simulink model "SM_smallScalePS"  (R2019a)
settings: Solver=ode23  StartTime=0.0  StopTime=5  RelTol=1e-3
undefined symbols (not defined in the file): D1, Delta
libraries: powerlib x9, sps_avr x1, spsHTGModel x1
settings Model: Creator=User  LastModifiedBy=User

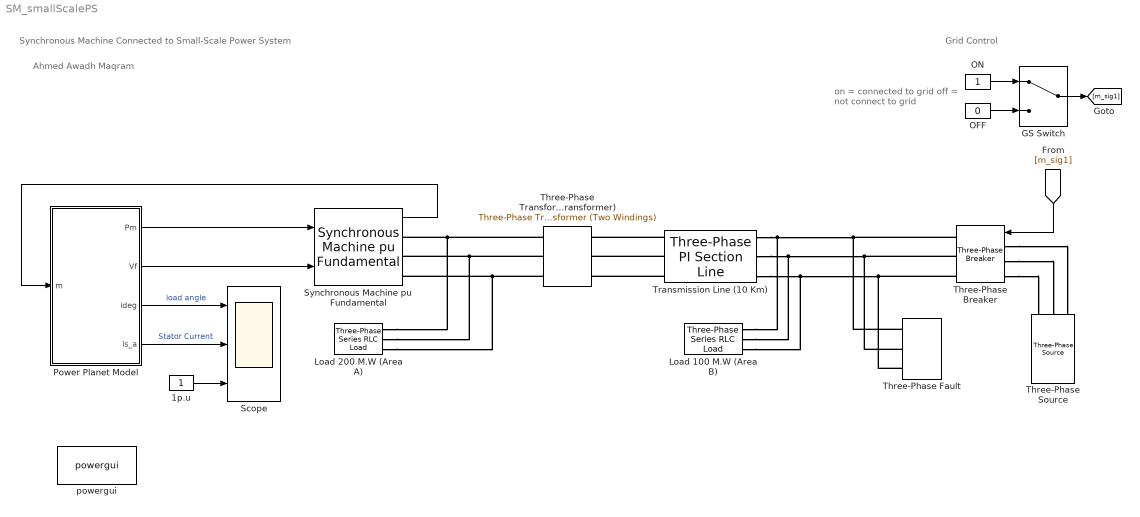
== system SM_smallScalePS ==
  note: Grid Control
  note: Synchronous Machine Connected to Small-Scale Power System
  note: Ahmed Awadh Maqram
  note: on = connected to grid
      | off = not connect to grid
  1p.u : Constant
  GS Switch : ManualSwitch
  Load 100 M.W (Area B) : powerlib/Elements/Three-Phase Series RLC Load  LConnTagsString=A|B|C  Configuration=Y (grounded)  NominalVoltage=230e3  Vabc=[1e3 1e3 1e3]  Vabcp=[1e3 1e3 1e3]  NominalFrequency=60  UnbalancedPower=off  ActivePower=100e6  InductivePower=0  CapacitivePower=0  Pabc=[10e3 9e3 11e3]  QLabc=[100 90 110]  QCabc=[100 90 110]  Pabcp=[10e3 9e3 11e3]  QLabcp=[100 90 110]  QCabcp=[100 90 110]  Measurements=None  LoadType=constant Z
      settings: SourceProductName=Simscape Electrical
  Load 200 M.W (Area A) : powerlib/Elements/Three-Phase Series RLC Load  LConnTagsString=A|B|C  Configuration=Y (grounded)  NominalVoltage=13.8e3  Vabc=[1e3 1e3 1e3]  Vabcp=[1e3 1e3 1e3]  NominalFrequency=60  UnbalancedPower=off  ActivePower=200e6  InductivePower=0  CapacitivePower=0  Pabc=[10e3 9e3 11e3]  QLabc=[100 90 110]  QCabc=[100 90 110]  Pabcp=[10e3 9e3 11e3]  QLabcp=[100 90 110]  QCabcp=[100 90 110]  Measurements=None  LoadType=constant Z
      settings: SourceProductName=Simscape Electrical
  OFF : Constant  Value=0
  ON : Constant
  Power Planet Model : Subsystem
  Scope : Scope  NumInputPorts=3
  Synchronous Machine pu Fundamental : powerlib/Machines/Synchronous Machine pu Fundamental  PresetModel=No  MechanicalLoad=Mechanical power Pm  ShowDetailedParameters=on  RotorType=Salient-pole  Units=per unit fundamental parameters  MeasurementBus=off  NominalParameters="[ 187E6  13800   60]"  Stator="[ 2.85E-03  0.114  1.19  0.36 ]"  Field="[ 5.79E-04  0.114]"  Dampers2=[0.0652, 0.5134, 0.0287, 0.2553, 7.765e-3, 0.9167 ]  Dampers1="[ 1.17E-02  0.182  1.97E-02  0.384 ]"  Mechanical=[ 3.7 0 20]  PolePairs=20  InitialConditions="[ 0  0  0  0  0  0  0  0  1 ]"  SetSaturation=off  Saturation=[0.6404,0.7127,0.8441,0.9214,0.9956,1.082,1.19,1.316,1.457;0.7,0.7698,0.8872,0.9466,0.9969,1.046,1.1,1.151,1.201]  LoadFlowParameters=[1,0,0,0,0]  TsPowergui=0  TsBlock=-1  IterativeModel=Trapezoidal non iterative  IterativeDiscreteModel=Trapezoidal non iterative  BusType=PV  Pref=0  Qref=0  Qmin=-inf  Qmax=inf  PLF=0  QLF=0
      settings: SourceProductName=Simscape Electrical  SourceProductBaseCode=PS
  Three-Phase Transformer (Step-up Transformer) : powerlib/Elements/Three-Phase Transformer (Two Windings)  Winding1Connection=Delta (D1)  Winding2Connection=Yg  CoreType=Three single-phase transformers  SetSaturation=off  Hysteresis=off  DataFile='hysteresis'  SetInitialFlux=off  Measurements=None  UNITS=pu  NominalPower=[ 250e6 , 60 ]  Winding1=[ 13.8e3 , 0.002 , 0.08 ]  Winding2=[ 230e3 , 0.002 , 0.08 ]  Rm=500  Lm=500  L0=0.5  Saturation=[ 0,0 ; 0.0024,1.2 ; 1.0,1.52 ]  InitialFluxes=[ 0.8 , -0.8 , 0.7 ]  BreakLoop=off  DiscreteSolver=Trapezoidal iterative  DataType=off  TransfoNumber=1
      settings: SourceProductName=Simscape Electrical
  Three-Phase Breaker : powerlib/Elements/Three-Phase Breaker  InitialState=open  SwitchA=on  SwitchB=on  SwitchC=on  SwitchTimes="[1/60  5/60]"  External=on  BreakerResistance=0.01  SnubberResistance=1e6  SnubberCapacitance=inf  Measurements=None
      settings: SourceProductName=Simscape Electrical
  Three-Phase Fault : powerlib/Elements/Three-Phase Fault  InitialStates=0  FaultA=on  FaultB=on  FaultC=on  GroundFault=on  SwitchTimes=[0.1 0.3]  External=off  SwitchStatus=NaN  FaultResistance=0.001  GroundResistance=0.01  SnubberResistance=1e6  SnubberCapacitance=inf  Measurements=None
      settings: SourceProductName=Simscape Electrical
  Three-Phase Source : powerlib/Electrical Sources/Three-Phase Source  InternalConnection=Yg  VoltagePhases=off  Voltage=230e3  PhaseAngle=0  Voltage_phases=[25e3 25e3 25e3]/sqrt(3)  PhaseAngles_phases=[0 -120 +120]  Frequency=60  NonIdealSource=on  SpecifyImpedance=off  Resistance=0.8929  Inductance=16.58e-3  ShortCircuitLevel=100e6  BaseVoltage=25e3  XRratio=7  BusType=swing  Pref=10e3  Qref=0  Prefabc=[10e3, 10e3, 10e3]  Qrefabc=[0, 0, 0]  Qmin=-inf  Qmax=inf
      settings: SourceProductName=Simscape Electrical
  Transmission Line (10 Km) : powerlib/Elements/Three-Phase PI Section Line  LConnTagsString=a|b|c  RConnTagsString=A|B|C  Frequency=60  Resistances=[ 0.01273 0.3864]  Inductances="[ 0.9337e-3  4.1264e-3]"  Capacitances=[12.74e-9 7.751e-9]  Length=10
      settings: SourceProductName=Simscape Electrical
  powergui : powerlib/powergui  Priority=1  SimulationMode=Phasor  SampleTime=50e-6  frequency=60  Iterations=50  frequencyindice=60  Pbase=100e6  ErrMax=1e-4  UnitsV=kV  UnitsW=MW  buscounter=0  FunctionMessages=off  echomessages=off  EnableUseOfTLC=off  CurrentSourceSwitches=off  DisableSnubberDevices=off  DisableRonSwitches=off  DisableVfSwitches=off  DisplayEquations=off  AutomaticDiscreteSolvers=off  SolverType=Tustin/Backward Euler (TBE)  Interpol=off  ExternalGateDelay=off  methode=off  Ts=100  x0status=blocks  SPID=on  SwTol=0  HookPort=off  NonlinearTolerance=0  nMaxIteration=15  ContinueOnMaxIteration=off  RestoreLinks=warning  ResistiveCurrentMeasurement=off  Frange=[0:2:500]  Ylog=off  Xlog=on  ShowGrid=off  save=off  variable=ZData  structure=0  ZoomFFT=off  StartTime=0.0  cycles=1  DisplayStyle=1  fundamental=60  FreqAxis=off  MaxFrequency=1000  frequencyindicesteady=1  RmsSteady=1  display=off
      settings: SourceProductName=Simscape Electrical
  wires:
  Power Planet Model/1(Pm) -> Synchronous Machine pu Fundamental/1
  Power Planet Model/2(Vf) -> Synchronous Machine pu Fundamental/2
  Synchronous Machine pu Fundamental/1 -> Power Planet Model/1(m)
  Power Planet Model/3(ideg) -> Scope/1  "load angle"
  Power Planet Model/4(is_a) -> Scope/2  "Stator Current"
  1p.u/1 -> Scope/3
  ON/1 -> GS Switch/1
  GS Switch/1 -> [m_sig1]
  OFF/1 -> GS Switch/2
  [m_sig1] -> Three-Phase Breaker/1
  connections:
  Three-Phase Transformer (Step-up Transformer)/LConn1 -- Synchronous Machine pu Fundamental/RConn1 -- Load 200 M.W (Area A)/LConn1
  Three-Phase Transformer (Step-up Transformer)/LConn2 -- Synchronous Machine pu Fundamental/RConn2 -- Load 200 M.W (Area A)/LConn2
  Three-Phase Transformer (Step-up Transformer)/LConn3 -- Synchronous Machine pu Fundamental/RConn3 -- Load 200 M.W (Area A)/LConn3
  Transmission Line (10 Km)/LConn1 -- Three-Phase Transformer (Step-up Transformer)/RConn1
  Transmission Line (10 Km)/LConn2 -- Three-Phase Transformer (Step-up Transformer)/RConn2
  Transmission Line (10 Km)/LConn3 -- Three-Phase Transformer (Step-up Transformer)/RConn3
  Transmission Line (10 Km)/RConn1 -- Load 100 M.W (Area B)/LConn1 -- Three-Phase Breaker/RConn1 -- Three-Phase Fault/LConn1
  Transmission Line (10 Km)/RConn2 -- Load 100 M.W (Area B)/LConn2 -- Three-Phase Breaker/RConn2 -- Three-Phase Fault/LConn2
  Transmission Line (10 Km)/RConn3 -- Load 100 M.W (Area B)/LConn3 -- Three-Phase Breaker/RConn3 -- Three-Phase Fault/LConn3
  Three-Phase Breaker/LConn1 -- Three-Phase Source/RConn1
  Three-Phase Breaker/LConn2 -- Three-Phase Source/RConn2
  Three-Phase Breaker/LConn3 -- Three-Phase Source/RConn3

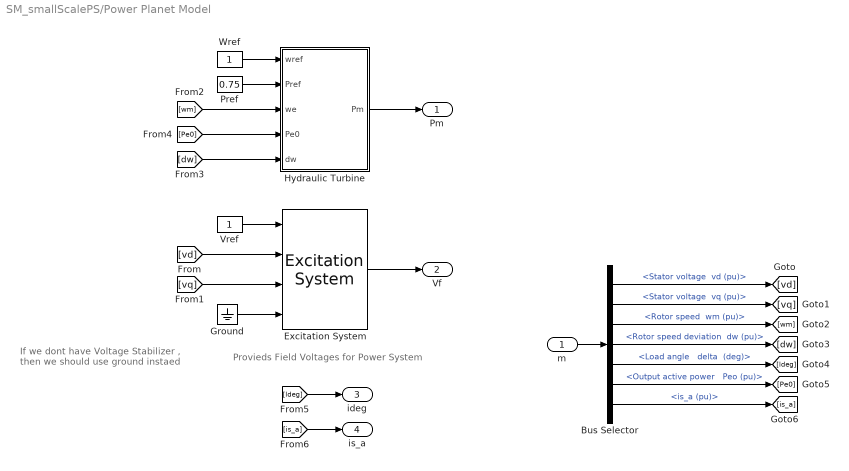
== system SM_smallScalePS/Power Planet Model ==
  note: Provieds Field Voltages for Power System
  note: If we dont have Voltage Stabilizer ,
      | then we should use ground instaed
  m : Inport
  Bus Selector : BusSelector  OutputSignals="dq0 components.Stator voltage  vd (pu),dq0 components.Stator voltage  vq (pu),Mechanical.Rotor speed  wm (pu),Mechanical.Rotor speed deviation  dw (pu),Load angle   delta  (deg),Output active power   Peo (pu),Stator current.is_a (pu)"
  Excitation System : sps_avr/Excitation System  tr=20e-3  reg=[ 300, 0.001 ]  exc=[ 1, 0 ]  tgr=[ 0, 0 ]  damp=[ 0.001, 0.1 ]  sat=[ 0, 0 ]  lim=[ -11.5, 11.5, 0 ]  v0="[1.0  1.28]"
      settings: SourceProductName=Simscape Electrical  SourceProductBaseCode=PS
  Ground : Ground
  Hydraulic Turbine : Subsystem  AncestorBlock=powerlib/Machines/Hydraulic Turbine and Governor  DialogController=POWERSYS.PowerSysDialog  mask(Hydraulic Turbine and Governor){sm=[ 10/3  0.07 ], gate=[  0.01  0.97518  -0.1  0.1 ], reg=[  0.05  1.163  0.105  0  0.01  ], hyd=[  0  2.67  ], dref=0, po=0.7516}
      mask prompts: sm "Servo-motor [ Ka()  Ta(sec) ]:"; gate "Gate opening limits [ gmin,gmax(pu)    vgmin,vgmax(pu/s) ]:"; reg "Permanent droop and regulator  [ Rp() Kp() Ki() Kd() Td(s) ]:"; hyd "Hydraulic turbine [ beta()  Tw(sec) ]:"; dref "Droop reference (0=power error, 1=gate opening):"; po "Initial mechanical power (pu):"
      mask help: Implements a hydraulic turbine combined to a PID governor system.
      mask init:
      | block = gcb;
      | [Ts, WantBlockChoice,ka,ta,gmin,gmax,vgmin,vgmax,Rp,Kp,ki,kd,td,beta,tw,go] = powericon('HydraulicTurbineInit',block,sm,gate,reg,hyd,po);
      | powericon('SetInternalModels','set',block,WantBlockChoice);
      settings: OpenFcn=sps_rtmsupport('OpenFcn',gcbh)
      mask Help: helpview(psbhelp);
      mask Display: disp('')
  Pref : Constant  Value=0.75
  Vref : Constant
  Wref : Constant
  Pm : Outport
  Vf : Outport  Port=2
  ideg : Outport  Port=3
  is_a : Outport  Port=4
  wires:
  Hydraulic Turbine/1(Pm) -> Pm/1
  Excitation System/1 -> Vf/1
  Ground/1 -> Excitation System/4
  Pref/1 -> Hydraulic Turbine/2(Pref)
  Wref/1 -> Hydraulic Turbine/1(wref)
  Vref/1 -> Excitation System/1
  m/1 -> Bus Selector/1
  Bus Selector/1 -> [vd]  "<Stator voltage  vd (pu)>"
  [vd] -> Excitation System/2
  Bus Selector/2 -> [vq]  "<Stator voltage  vq (pu)>"
  Bus Selector/3 -> [wm]  "<Rotor speed  wm (pu)>"
  Bus Selector/4 -> [dw]  "<Rotor speed deviation  dw (pu)>"
  Bus Selector/5 -> [ldeg]  "<Load angle   delta  (deg)>"
  Bus Selector/6 -> [Pe0]  "<Output active power   Peo (pu)>"
  Bus Selector/7 -> [is_a]  "<is_a (pu)>"
  [vq] -> Excitation System/3
  [wm] -> Hydraulic Turbine/3(we)
  [dw] -> Hydraulic Turbine/5(dw)
  [Pe0] -> Hydraulic Turbine/4(Pe0)
  [ldeg] -> ideg/1
  [is_a] -> is_a/1

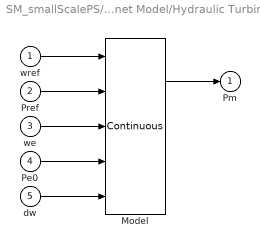
== system SM_smallScalePS/Power Planet Model/Hydraulic Turbine ==
  wref : Inport
  Pref : Inport  Port=2
  we : Inport  Port=3
  Pe0 : Inport  Port=4
  dw : Inport  Port=5
  Model : spsHTGModel/Continuous  sm=sm  gate=gate  reg=reg  hyd=hyd  dref=dref  po=po
      settings: SourceProductName=Simscape Electrical  SourceProductBaseCode=PS
  Pm : Outport  InitialOutput=0
  wires:
  Model/1 -> Pm/1
  dw/1 -> Model/5
  Pe0/1 -> Model/4
  we/1 -> Model/3
  Pref/1 -> Model/2
  wref/1 -> Model/1
